simulink library "lookUpGaitDynamics"  (R2016b)
settings: Solver=VariableStepAuto  StartTime=0.0  StopTime=10.0  RelTol=1e-3
libraries: simulink_extras x1
settings Model: Creator=march  LastModifiedBy=Taeke

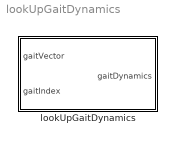
== system lookUpGaitDynamics ==
  lookUpGaitDynamics : Subsystem

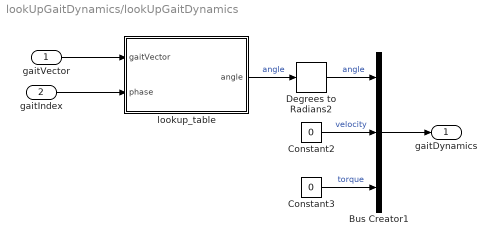
== system lookUpGaitDynamics/lookUpGaitDynamics ==
  gaitVector : Inport
  gaitIndex : Inport  Port=2
  Bus Creator1 : BusCreator  Inputs=3  OutDataTypeStr=Bus: JointDynamics  NonVirtualBus=on
  Constant2 : Constant  Value=0
  Constant3 : Constant  Value=0
  Degrees to Radians2 : simulink_extras/Transformations/Degrees to Radians
  lookup_table : MATLAB Function  TreatAsAtomicUnit=on
  gaitDynamics : Outport  OutDataTypeStr=Bus: JointDynamics
  wires:
  gaitIndex/1 -> lookup_table/2(phase)
  Constant2/1 -> Bus Creator1/2  "velocity"
  Degrees to Radians2/1 -> Bus Creator1/1  "angle"
  lookup_table/1(angle) -> Degrees to Radians2/1  "angle"
  Constant3/1 -> Bus Creator1/3  "torque"
  Bus Creator1/1 -> gaitDynamics/1
  gaitVector/1 -> lookup_table/1(gaitVector)

== matlab function lookUpGaitDynamics/lookup_table ==
  data: gaitVector input; angle output; phase input
function angle  = lookup_table(gaitVector, phase)
% wrapper for lookup_table
[angle] = lookup_table(gaitVector, phase);
end
